simulink model "dashboard_ex"  (R2022b)
settings: Solver=FixedStepAuto  StartTime=0.0  StopTime=100  FixedStep=1  RelTol=1e-3
settings Model: SimulationMode=accelerator  PacingRate=3  Creator=Brigosha_Guest  LastModifiedBy=Brigosha_Guest

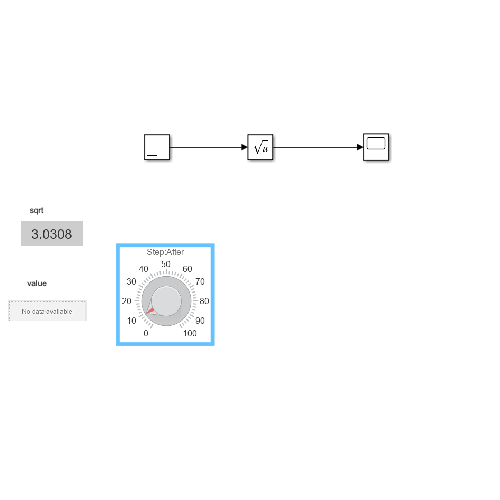
[thumbnail: Simulink's stored preview of the top-level diagram]
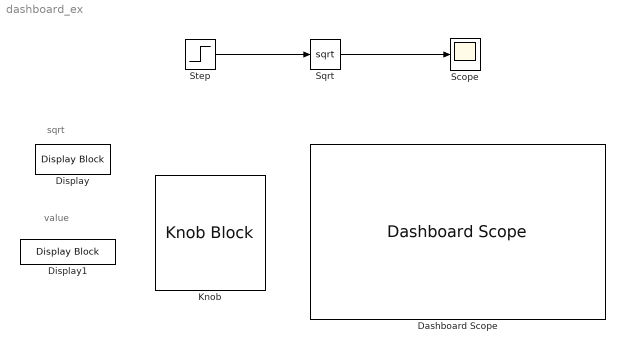
== system dashboard_ex ==
  note: sqrt
  note: value
  Dashboard Scope : DashboardScope  Ymin=-1  Ymax=100  ScaleAtStop=off  UpdateMode=Scroll
  Display : DisplayBlock  LabelPosition=Hide  Transparency=1  Layout=Fill available space
  Display1 : DisplayBlock  LabelPosition=Hide  Transparency=1
  Knob : KnobBlock
  Scope : Scope
  Sqrt : Sqrt
  Step : Step  After=9.18547503153483  SampleTime=0
  wires:
  Step/1 -> Sqrt/1
  Sqrt/1 -> Scope/1
